simulink library "VehicleBody"  (R2023b)
settings: Solver=VariableStepAuto  StartTime=0.0  StopTime=10.0  RelTol=1e-3
values from neighbouring files (symbols this model uses):
  f_r = 0.4    [init_model_opti.m]    (also in run_EV_PT_2spd.m)
  g = 9.81    [init_model_opti.m]    (also in run_EV_PT_2spd.m)
  rho = 1.18    [init_model_opti.m]    (also in run_EV_PT_2spd.m)
undefined symbols (not defined in the file or in its folder): h, r_wheel
settings Model: Creator=dadikozyanaa  LastModifiedBy=koenjacobs
settings DebuggingCC: UnconnectedInputMsg=warning  UnconnectedOutputMsg=warning  UnconnectedLineMsg=warning
settings ModelReferenceCC: EnableRefExpFcnMdlSchedulingChecks=on
settings RTWCC: DLArmComputeVersion=19.05

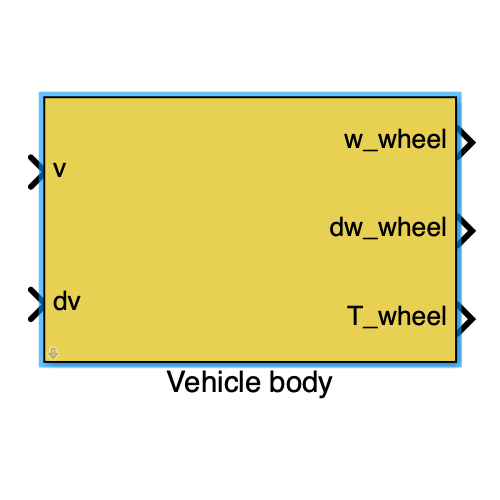
[thumbnail: Simulink's stored preview of the top-level diagram]
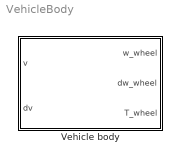
== system VehicleBody ==
  Vehicle body : Subsystem  mask(Vehicle body){drivetype=FWD, m_f=750, mt2m_f=5, A_f=1.8, d_wheel=0.5, cw=0.22, mu=0.008}
      mask prompts: drivetype "Drivetrain type"; m_f "Total vehicle mass [kg]:"; mt2m_f "Rotating mass [%]:"; A_f "Vehicle cross section [m2]:"; d_wheel "Wheel diameter [m]:"; cw "Air drag coefficient [-]:"; mu "Rolling resistance coefficient [-]:"
      mask help:
      | This block computes the power required from the vehicle.
      |
      | Input:
      | =====
      | 	v	Speed [m/s]
      | 	dv	Acceleration [m/s^2]
      | 	slope	Road slope [rad] (optional)
      |
      | Output:
      | ======
      | 	w_wheel	Speed of the wheel [rad/s]
      | 	dw_wheel	Acceleration of the wheel [rad/s^2]
      | 	T_wheel	Torque on the wheel [Nm]
      |
      | Drivetrain type:
      | =====
      | Affects the Regen Brake Factor [-] :
      |
      |        FWD --> F_r = 0.6
      |        RWD --> F_r = 0.4
      |        AWD --> F_r = 0.9
      mask init:
      | init_vehicle;
      mask TypeOptions drivetype: FWD | RWD | AWD

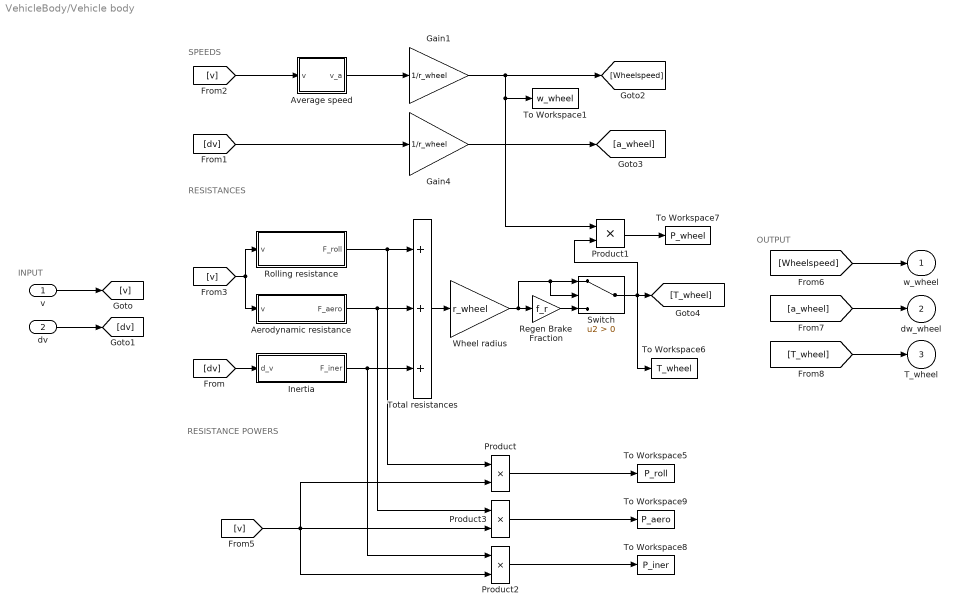
== system VehicleBody/Vehicle body ==
  note: OUTPUT
  note: SPEEDS
  note: RESISTANCE POWERS
  note: RESISTANCES
  note: INPUT
  v : Inport
  dv : Inport  Port=2
  Aerodynamic resistance : Subsystem
  Average speed : Subsystem
  Gain1 : Gain  Gain=1/r_wheel  SaturateOnIntegerOverflow=on  OutDataTypeStr=Inherit: Same as input  ParamDataTypeStr=Inherit: Same as input
  Gain4 : Gain  Gain=1/r_wheel  SaturateOnIntegerOverflow=on  OutDataTypeStr=Inherit: Same as input  ParamDataTypeStr=Inherit: Same as input
  Inertia : Subsystem
  Product : Product  InputSameDT=on  RndMeth=Zero  SaturateOnIntegerOverflow=on  OutDataTypeStr=Inherit: Same as first input
  Product1 : Product
  Product2 : Product  InputSameDT=on  RndMeth=Zero  SaturateOnIntegerOverflow=on  OutDataTypeStr=Inherit: Same as first input
  Product3 : Product  InputSameDT=on  RndMeth=Zero  SaturateOnIntegerOverflow=on  OutDataTypeStr=Inherit: Same as first input
  Regen Brake Fraction : Gain  Gain=f_r
  Rolling resistance : Subsystem
  Switch : Switch  Criteria=u2 > Threshold  SaturateOnIntegerOverflow=off  InputSameDT=off
  To Workspace1 : ToWorkspace  VariableName=w_wheel  SampleTime=-1
  To Workspace5 : ToWorkspace  VariableName=P_roll  SampleTime=-1
  To Workspace6 : ToWorkspace  VariableName=T_wheel  SampleTime=-1
  To Workspace7 : ToWorkspace  VariableName=P_wheel  SampleTime=-1
  To Workspace8 : ToWorkspace  VariableName=P_iner  SampleTime=-1
  To Workspace9 : ToWorkspace  VariableName=P_aero  SampleTime=-1
  Total resistances : Sum  Inputs=+++  InputSameDT=on  SaturateOnIntegerOverflow=on  OutDataTypeStr=Inherit: Same as first input
  Wheel radius : Gain  Gain=r_wheel  SaturateOnIntegerOverflow=on  OutDataTypeStr=Inherit: Same as input  ParamDataTypeStr=Inherit: Same as input
  w_wheel : Outport  InitialOutput=0
  dw_wheel : Outport  Port=2  InitialOutput=0
  T_wheel : Outport  Port=3  InitialOutput=0
  wires:
  dv/1 -> [dv]
  Inertia/1(F_iner) -> Product2/1, Total resistances/3
  Rolling resistance/1(F_roll) -> Product/1, Total resistances/1
  [v] -> Aerodynamic resistance/1(v), Rolling resistance/1(v)
  [v] -> Product2/2, Product3/2, Product/2
  [v] -> Average speed/1(v)
  Aerodynamic resistance/1(F_aero) -> Product3/1, Total resistances/2
  Wheel radius/1 -> Switch/1, Switch/2, Regen Brake Fraction/1
  Product/1 -> To Workspace5/1
  Total resistances/1 -> Wheel radius/1
  [dv] -> Gain4/1
  Gain4/1 -> [a_wheel]
  Average speed/1(v_a) -> Gain1/1
  Product2/1 -> To Workspace8/1
  v/1 -> [v]
  Product3/1 -> To Workspace9/1
  Gain1/1 -> Product1/1, To Workspace1/1, [Wheelspeed]
  [dv] -> Inertia/1(d_v)
  Regen Brake Fraction/1 -> Switch/3
  Switch/1 -> Product1/2, [T_wheel], To Workspace6/1
  [Wheelspeed] -> w_wheel/1
  [a_wheel] -> dw_wheel/1
  [T_wheel] -> T_wheel/1
  Product1/1 -> To Workspace7/1

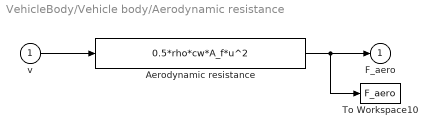
== system VehicleBody/Vehicle body/Aerodynamic resistance ==
  v : Inport
  Aerodynamic resistance : Fcn  Expr=0.5*rho*cw*A_f*u^2
  To Workspace10 : ToWorkspace  VariableName=F_aero  SampleTime=-1
  F_aero : Outport  InitialOutput=0
  wires:
  v/1 -> Aerodynamic resistance/1
  Aerodynamic resistance/1 -> F_aero/1, To Workspace10/1

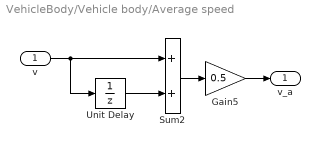
== system VehicleBody/Vehicle body/Average speed ==
  v : Inport
  Gain5 : Gain  Gain=0.5  SaturateOnIntegerOverflow=on  OutDataTypeStr=Inherit: Same as input  ParamDataTypeStr=Inherit: Same as input
  Sum2 : Sum  InputSameDT=on  SaturateOnIntegerOverflow=on  OutDataTypeStr=Inherit: Same as first input
  Unit Delay : UnitDelay  SampleTime=h
  v_a : Outport  InitialOutput=0
  wires:
  Unit Delay/1 -> Sum2/2
  Sum2/1 -> Gain5/1
  Gain5/1 -> v_a/1
  v/1 -> Sum2/1, Unit Delay/1

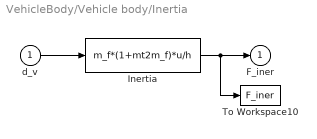
== system VehicleBody/Vehicle body/Inertia ==
  d_v : Inport
  Inertia : Fcn  Expr=m_f*(1+mt2m_f)*u/h
  To Workspace10 : ToWorkspace  VariableName=F_iner  SampleTime=-1
  F_iner : Outport  InitialOutput=0
  wires:
  Inertia/1 -> F_iner/1, To Workspace10/1
  d_v/1 -> Inertia/1

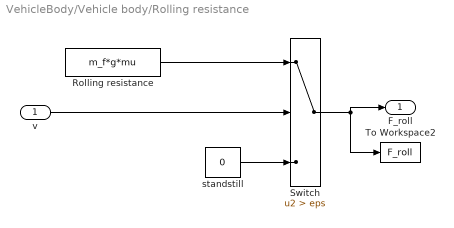
== system VehicleBody/Vehicle body/Rolling resistance ==
  v : Inport
  Rolling resistance : Constant  Value=m_f*g*mu
  Switch : Switch  Criteria=u2 > Threshold  Threshold=eps  SaturateOnIntegerOverflow=off  InputSameDT=off
  To Workspace2 : ToWorkspace  VariableName=F_roll  SampleTime=-1
  standstill : Constant  Value=0
  F_roll : Outport
  wires:
  Switch/1 -> To Workspace2/1, F_roll/1
  v/1 -> Switch/2
  standstill/1 -> Switch/3
  Rolling resistance/1 -> Switch/1
